simulink model "Simulation1"  (R2021a)
settings: Solver=VariableStepAuto  StartTime=0.0  StopTime=10.0  RelTol=1e-3
values from neighbouring files (symbols this model uses):
  Fp = 100    [ModelVisualisation.m]
  g = 9.81    [ModelVisualisation.m]    (also in Test.m)
  If = [Ixx 0 0;0 Iyy 0;0 0 Izz]    [ModelVisualisation.m]
  Kpm = mc/Ip    (= 0.005)    [ModelVisualisation.m]
  KVarianceBruit = 10    [ModelVisualisation.m]
  KVarianceBruiVent = 10    [ModelVisualisation.m]
  mi = 7    [ModelVisualisation.m]
  PhiRafale = pi/4    (= 0.785398163397)    [ModelVisualisation.m]
  Rafale = 5    [ModelVisualisation.m]
  SrefAA = LongueurAA*(CsaumonAA+CemplentureAA)/2    (= 0.02805)    [ModelVisualisation.m]
  SrefAC = LongueurAC*(CsaumonAC+CemplentureAC)/2    (= 0.002)    [ModelVisualisation.m]
  SrefC = 1/3*ZCC*2*pi*RayonCC    (= 0.0502654824574)    [ModelVisualisation.m]
  SrefCC = LongueurCC*pi*2*RayonCC    (= 1.25663706144)    [ModelVisualisation.m]
  TBruitP = 0.1    [ModelVisualisation.m]
  TBruitVent = 0.2    [ModelVisualisation.m]
  TDebutRafale = 2    [ModelVisualisation.m]
  TempsRafale = 0.7    [ModelVisualisation.m]
  Tpropultion = 2    [ModelVisualisation.m]
  VarianceBruitP = 1    [ModelVisualisation.m]
  VarianceBruitVent = 2    [ModelVisualisation.m]
settings Model: Creator=Adhemar  LastModifiedBy=adhem

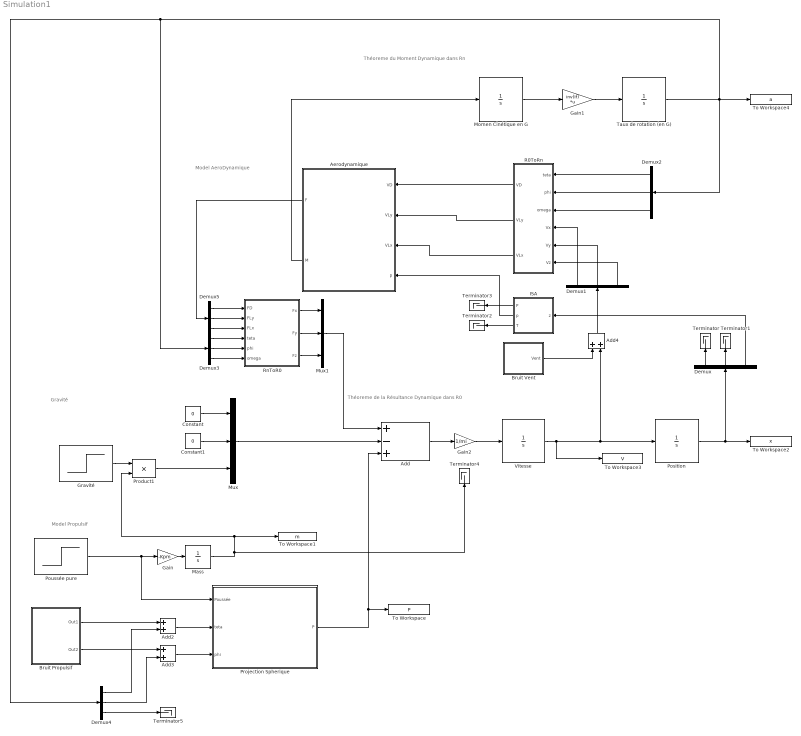
== system Simulation1 ==
  note: Théoreme du Moment Dynamique dans Rn
  note: Théoreme de la Résultance Dynamique dans R0
  note: Model AeroDynamique
  note: Gravité
  note: Model Propulsif
  Add : Sum  Inputs=+-+
  Add2 : Sum
  Add3 : Sum
  Add4 : Sum
  Aerodynamique : Subsystem
  Bruit Propulsif : Subsystem
  Bruit Vent : Subsystem
  Constant : Constant  Value=0
  Constant1 : Constant  Value=0
  Demux{,1..5} (6 alike) : Demux  Outputs=3
  Gain : Gain  Gain=-Kpm
  Gain1 : Gain  Gain=inv(If)  Multiplication=Matrix(K*u)
  Gain2 : Gain  Gain=1/mi
  Gravité : Step  Time=0  Before=g  After=g  SampleTime=0
  ISA : MATLAB Function  TreatAsAtomicUnit=on
  Mass : Integrator  InitialCondition=mi
  Momen Cinétique en G : Integrator
  Mux : Mux  Inputs=3
  Mux1 : Mux  Inputs=3
  Position : Integrator  InitialCondition=[0,0,0]
  Poussée pure : Step  Time=Tpropultion  Before=Fp  After=0  SampleTime=0
  Product1 : Product
  Projection Spherique : Subsystem
  R0ToRn : MATLAB Function  TreatAsAtomicUnit=on
  RnToR0 : MATLAB Function  TreatAsAtomicUnit=on
  Taux de rotation (en G) : Integrator
  Terminator{,1..5} (6 alike) : Terminator
  To Workspace : ToWorkspace  VariableName=P  SaveFormat=Timeseries  SampleTime=-1
  To Workspace1 : ToWorkspace  VariableName=m  SaveFormat=Timeseries  SampleTime=-1
  To Workspace2 : ToWorkspace  VariableName=x  SaveFormat=Timeseries  SampleTime=-1
  To Workspace3 : ToWorkspace  VariableName=V  SaveFormat=Timeseries  SampleTime=-1
  To Workspace4 : ToWorkspace  VariableName=a  SaveFormat=Timeseries  SampleTime=-1
  Vitesse : Integrator  InitialCondition=[0,0,0]
  wires:
  Add/1 -> Gain2/1
  Poussée pure/1 -> Gain/1, Projection Spherique/1(Poussée)
  Projection Spherique/1(P) -> Add/3, To Workspace/1
  Gravité/1 -> Product1/1
  Gain2/1 -> Vitesse/1
  Mass/1 -> Terminator4/1, To Workspace1/1, Product1/2
  Gain/1 -> Mass/1
  Product1/1 -> Mux/3
  Position/1 -> To Workspace2/1, Demux/1
  Bruit Propulsif/1(Out1) -> Add2/1
  Bruit Propulsif/2(Out2) -> Add3/1
  Mux1/1 -> Add/1
  Constant/1 -> Mux/1
  Mux/1 -> Add/2
  Constant1/1 -> Mux/2
  Demux/3 -> ISA/1(z)
  Demux/1 -> Terminator/1
  Demux/2 -> Terminator1/1
  Demux1/1 -> R0ToRn/4(Vx)
  Vitesse/1 -> Position/1, Add4/2, To Workspace3/1
  Demux1/3 -> R0ToRn/6(Vz)
  Demux1/2 -> R0ToRn/5(Vy)
  Momen Cinétique en G/1 -> Gain1/1
  Gain1/1 -> Taux de rotation (en G)/1
  Add2/1 -> Projection Spherique/2(teta)
  Add3/1 -> Projection Spherique/3(phi)
  Add4/1 -> Demux1/1
  Bruit Vent/1(Vent) -> Add4/1
  Demux2/3 -> R0ToRn/3(omega)
  Demux2/2 -> R0ToRn/2(phi)
  Demux2/1 -> R0ToRn/1(teta)
  RnToR0/1(Fx) -> Mux1/1
  RnToR0/2(Fy) -> Mux1/2
  RnToR0/3(Fz) -> Mux1/3
  Demux3/1 -> RnToR0/4(teta)
  Demux3/2 -> RnToR0/5(phi)
  Demux3/3 -> RnToR0/6(omega)
  Taux de rotation (en G)/1 -> Demux2/1, Demux4/1, Demux3/1, To Workspace4/1
  ISA/3(T) -> Terminator2/1
  ISA/1(P) -> Terminator3/1
  Demux4/1 -> Add2/2
  Demux4/2 -> Add3/2
  Demux4/3 -> Terminator5/1
  Aerodynamique/2(M) -> Momen Cinétique en G/1
  R0ToRn/1(VD) -> Aerodynamique/1(VD)
  R0ToRn/2(VLy) -> Aerodynamique/2(VLy)
  R0ToRn/3(VLx) -> Aerodynamique/3(VLx)
  ISA/2(p) -> Aerodynamique/4(p)
  Aerodynamique/1(F) -> Demux5/1
  Demux5/1 -> RnToR0/1(FD)
  Demux5/2 -> RnToR0/2(FLy)
  Demux5/3 -> RnToR0/3(FLx)

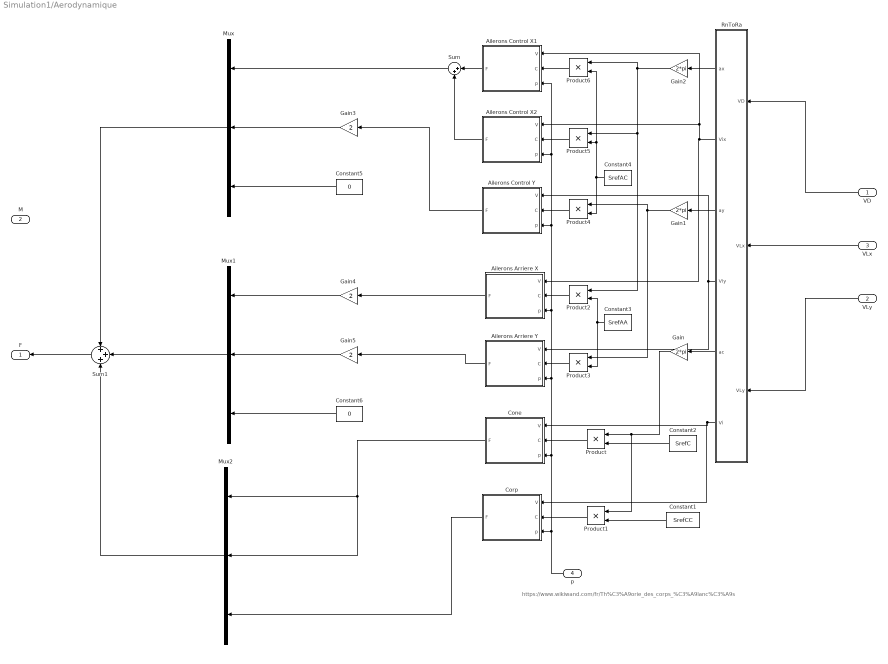
== system Simulation1/Aerodynamique ==
  note: https://www.wikiwand.com/fr/Th%C3%A9orie_des_corps_%C3%A9lanc%C3%A9s
  VD : Inport
  VLy : Inport  Port=2
  VLx : Inport  Port=3
  p : Inport  Port=4
  Ailerons Arriere X : MATLAB Function  TreatAsAtomicUnit=on
  Ailerons Arriere Y : MATLAB Function  TreatAsAtomicUnit=on
  Ailerons Control X1 : MATLAB Function  TreatAsAtomicUnit=on
  Ailerons Control X2 : MATLAB Function  TreatAsAtomicUnit=on
  Ailerons Control Y : MATLAB Function  TreatAsAtomicUnit=on
  Cone : MATLAB Function  TreatAsAtomicUnit=on
  Constant1 : Constant  Value=SrefCC
  Constant2 : Constant  Value=SrefC
  Constant3 : Constant  Value=SrefAA
  Constant4 : Constant  Value=SrefAC
  Constant5 : Constant  Value=0
  Constant6 : Constant  Value=0
  Corp : MATLAB Function  TreatAsAtomicUnit=on
  Gain : Gain  Gain=2*pi
  Gain1 : Gain  Gain=2*pi
  Gain2 : Gain  Gain=2*pi
  Gain3 : Gain  Gain=2
  Gain4 : Gain  Gain=2
  Gain5 : Gain  Gain=2
  Mux : Mux  Inputs=3
  Mux1 : Mux  Inputs=3
  Mux2 : Mux  Inputs=3
  Product{,1..6} (7 alike) : Product
  RnToRa : MATLAB Function  TreatAsAtomicUnit=on
  Sum : Sum  Inputs=|++
  Sum1 : Sum  Inputs=+++
  F : Outport
  M : Outport  Port=2
  wires:
  VLy/1 -> RnToRa/3(VLy)
  p/1 -> Ailerons Control Y/3(p), Ailerons Control X2/3(p), Ailerons Control X1/3(p), Ailerons Arriere X/3(p), Ailerons Arriere Y/3(p), Cone/3(p), Corp/3(p)
  Constant2/1 -> Product/2
  Corp/1(F) -> Mux2/3
  VLx/1 -> RnToRa/2(VLx)
  VD/1 -> RnToRa/1(VD)
  Ailerons Arriere X/1(F) -> Gain4/1
  Cone/1(F) -> Mux2/2, Mux2/1
  RnToRa/1(ax) -> Gain2/1
  RnToRa/5(ac) -> Gain/1
  Gain/1 -> Product1/1, Product/1
  Product/1 -> Cone/2(C)
  Constant1/1 -> Product1/2
  Product1/1 -> Corp/2(C)
  RnToRa/6(Vi) -> Cone/1(V), Corp/1(V)
  RnToRa/3(ay) -> Gain1/1
  Gain2/1 -> Product5/1, Product2/1, Product6/1
  Product2/1 -> Ailerons Arriere X/2(C)
  Product3/1 -> Ailerons Arriere Y/2(C)
  Gain1/1 -> Product3/1, Product4/1
  Constant3/1 -> Product2/2, Product3/2
  Product4/1 -> Ailerons Control Y/2(C)
  Product5/1 -> Ailerons Control X2/2(C)
  Product6/1 -> Ailerons Control X1/2(C)
  Constant4/1 -> Product5/2, Product6/2, Product4/2
  Sum/1 -> Mux/1
  Ailerons Control X1/1(F) -> Sum/1
  Ailerons Control X2/1(F) -> Sum/2
  Ailerons Control Y/1(F) -> Gain3/1
  Gain3/1 -> Mux/2
  Constant5/1 -> Mux/3
  Gain4/1 -> Mux1/1
  Constant6/1 -> Mux1/3
  Ailerons Arriere Y/1(F) -> Gain5/1
  Gain5/1 -> Mux1/2
  RnToRa/4(Viy) -> Ailerons Control Y/1(V), Ailerons Arriere Y/1(V)
  RnToRa/2(Vix) -> Ailerons Arriere X/1(V), Ailerons Control X1/1(V), Ailerons Control X2/1(V)
  Sum1/1 -> F/1
  Mux1/1 -> Sum1/2
  Mux2/1 -> Sum1/3
  Mux/1 -> Sum1/1

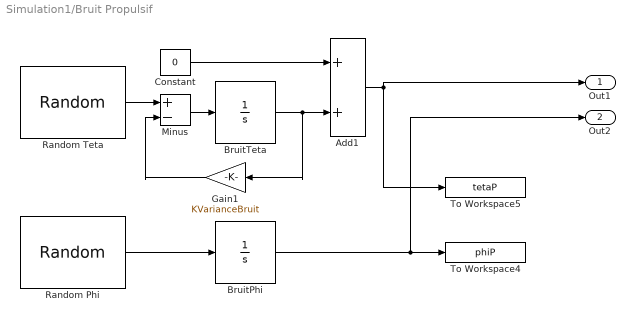
== system Simulation1/Bruit Propulsif ==
  Add1 : Sum
  BruitPhi : Integrator
  BruitTeta : Integrator
  Constant : Constant  Value=0
  Gain1 : Gain  Gain=KVarianceBruit
  Minus : Sum  Inputs=+-
  Random Phi : RandomNumber  Variance=VarianceBruitP  SampleTime=TBruitP
  Random Teta : RandomNumber  Variance=VarianceBruitP  Seed=1  SampleTime=TBruitP
  To Workspace4 : ToWorkspace  VariableName=phiP  SaveFormat=Timeseries  SampleTime=-1
  To Workspace5 : ToWorkspace  VariableName=tetaP  SaveFormat=Timeseries  SampleTime=-1
  Out1 : Outport
  Out2 : Outport  Port=2
  wires:
  Minus/1 -> BruitTeta/1
  BruitPhi/1 -> Out2/1, To Workspace4/1
  BruitTeta/1 -> Gain1/1, Add1/2
  Random Phi/1 -> BruitPhi/1
  Add1/1 -> Out1/1, To Workspace5/1
  Random Teta/1 -> Minus/1
  Gain1/1 -> Minus/2
  Constant/1 -> Add1/1

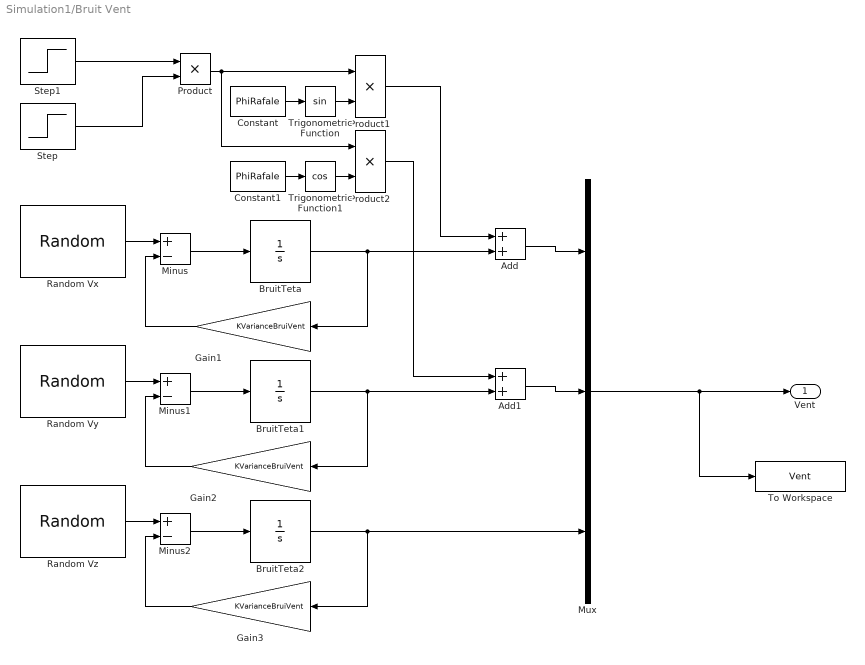
== system Simulation1/Bruit Vent ==
  Add : Sum
  Add1 : Sum
  BruitTeta : Integrator
  BruitTeta1 : Integrator
  BruitTeta2 : Integrator
  Constant : Constant  Value=PhiRafale
  Constant1 : Constant  Value=PhiRafale
  Gain1 : Gain  Gain=KVarianceBruiVent
  Gain2 : Gain  Gain=KVarianceBruiVent
  Gain3 : Gain  Gain=KVarianceBruiVent
  Minus : Sum  Inputs=+-
  Minus1 : Sum  Inputs=+-
  Minus2 : Sum  Inputs=+-
  Mux : Mux  Inputs=3
  Product : Product
  Product1 : Product
  Product2 : Product
  Random Vx : RandomNumber  Variance=VarianceBruitVent  SampleTime=TBruitVent
  Random Vy : RandomNumber  Variance=VarianceBruitVent  Seed=1  SampleTime=TBruitVent
  Random Vz : RandomNumber  Variance=VarianceBruitVent  Seed=2  SampleTime=TBruitVent
  Step : Step  Time=TDebutRafale  After=Rafale  SampleTime=0
  Step1 : Step  Time=TDebutRafale+TempsRafale  Before=1  After=0  SampleTime=0
  To Workspace : ToWorkspace  VariableName=Vent  SaveFormat=Timeseries  SampleTime=-1
  Trigonometric Function : Trigonometry
  Trigonometric Function1 : Trigonometry  Operator=cos
  Vent : Outport
  wires:
  Minus/1 -> BruitTeta/1
  BruitTeta/1 -> Add/2, Gain1/1
  Random Vx/1 -> Minus/1
  Gain1/1 -> Minus/2
  Mux/1 -> To Workspace/1, Vent/1
  Gain2/1 -> Minus1/2
  Minus1/1 -> BruitTeta1/1
  BruitTeta1/1 -> Add1/2, Gain2/1
  Random Vy/1 -> Minus1/1
  Minus2/1 -> BruitTeta2/1
  Random Vz/1 -> Minus2/1
  Gain3/1 -> Minus2/2
  BruitTeta2/1 -> Mux/3, Gain3/1
  Step/1 -> Product/2
  Step1/1 -> Product/1
  Product/1 -> Product2/1, Product1/1
  Add/1 -> Mux/1
  Product1/1 -> Add/1
  Trigonometric Function/1 -> Product1/2
  Constant/1 -> Trigonometric Function/1
  Add1/1 -> Mux/2
  Constant1/1 -> Trigonometric Function1/1
  Trigonometric Function1/1 -> Product2/2
  Product2/1 -> Add1/1

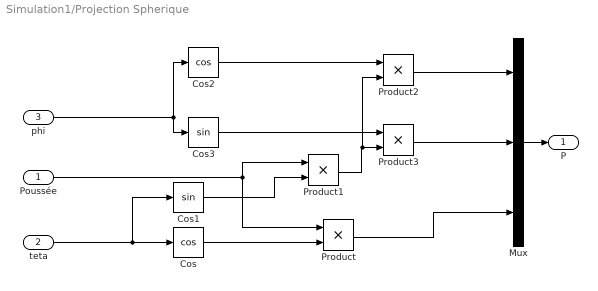
== system Simulation1/Projection Spherique ==
  Poussée : Inport
  teta : Inport  Port=2
  phi : Inport  Port=3
  Cos : Trigonometry  Operator=cos
  Cos1 : Trigonometry
  Cos2 : Trigonometry  Operator=cos
  Cos3 : Trigonometry
  Mux : Mux  Inputs=3
  Product{,1..3} (4 alike) : Product
  P : Outport
  wires:
  Poussée/1 -> Product1/1, Product/1
  Cos/1 -> Product/2
  teta/1 -> Cos1/1, Cos/1
  Product/1 -> Mux/3
  Cos1/1 -> Product1/2
  phi/1 -> Cos3/1, Cos2/1
  Product2/1 -> Mux/1
  Product3/1 -> Mux/2
  Product1/1 -> Product2/2, Product3/2
  Cos3/1 -> Product3/1
  Cos2/1 -> Product2/1
  Mux/1 -> P/1

== matlab function Simulation1/Aerodynamique/Ailerons Arriere Y ==
  data: V input; C input; p input; F output
function F = VToFAero(V,C,p)
    F=0.5*p*C*V^2;
end

== matlab function Simulation1/Aerodynamique/Ailerons Control X2 ==
  data: V input; C input; p input; F output
function F = VToFAero(V,C,p)
    F=0.5*p*C*V^2;
end

== matlab function Simulation1/Aerodynamique/Ailerons Control Y ==
  data: V input; C input; p input; F output
function F = VToFAero(V,C,p)
    F=0.5*p*C*V^2;
end

== matlab function Simulation1/R0ToRn ==
  data: teta input; phi input; omega input; Vx input; VD output; VLy output; Vy input; Vz input; VLx output
function [VD,VLy,VLx] = ChangementBase(teta,phi,omega,Vx,Vy,Vz)
    V=sqrt(Vx^2+Vy^2+Vz^2);
    
    %Changement base B
    VBx=cos(phi)*Vx+sin(phi)*Vy;
    VBy=cos(phi)*Vy-sin(phi)*Vx;
    VBz=Vz;
    %Changement base A
    VAx=VBx;
    VAy=cos(teta)*VBy+sin(teta)*VBz;
    VAz=cos(teta)*VBz-sin(teta)*VBy;
    %Changement base Aérodynamique
    VD=VAz;
    VLx=VAx*cos(omega)+VAy*sin(omega);
    VLy=VAy*cos(omega)-VAx*sin(omega);
    
    
    
    % A faire sous forme de matrice de passage
end

== matlab function Simulation1/ISA ==
  data: z input; P output; p output; T output

function [P,p,T]=ISA(z)
    
    g=9.81;
    r=287.04; %Constante des gaz parfait air (J/Kg/K)
    T0=287.15; %Température au sol A regler avant le lancement (K)
    Tz=-0.0065; %(K)
    P0=101325; %Pression au sol à regler avant le lancement (pa)
    p0=P0/(r*T0); %Densité de l'air (Kg/m3) 
    
    T=double(T0+Tz*z);
    P=double(P0*(1+(Tz/T0)*z)^(-g/(r*Tz)));
    p=double(P/(r*T));
end

== matlab function Simulation1/RnToR0 ==
  data: FD input; Fx output; FLy input; FLx input; teta input; phi input; omega input; Fy output; Fz output
function [Fx,Fy,Fz] = ChangeBase(FD,FLy,FLx,teta,phi,omega)
    Fx=0;
    Fy=0;
    Fz=0;
end

== matlab function Simulation1/Aerodynamique/Cone ==
  data: V input; C input; p input; F output
function F = VToFAero(V,C,p)
    F=0.5*p*C*V^2;
end

== matlab function Simulation1/Aerodynamique/Corp ==
  data: V input; C input; p input; F output
function F = VToFAero(V,C,p)
    F=0.5*p*C*V^2;
end

== matlab function Simulation1/Aerodynamique/Ailerons Arriere X ==
  data: V input; C input; p input; F output
function F = VToFAero(V,C,p)
    F=0.5*p*C*V^2;
end

== matlab function Simulation1/Aerodynamique/Ailerons Control X1 ==
  data: V input; C input; p input; F output
function F = VToFAero(V,C,p)
    F=0.5*p*C*V^2;
end

== matlab function Simulation1/Aerodynamique/RnToRa ==
  data: VD input; ax output; VLx input; VLy input; Vix output; ay output; Viy output; ac output; Vi output
function [ax,Vix,ay,Viy,ac,Vi] = ChangeBase(VD,VLx,VLy)
    
    ax=atan(VLx/VD);
    Vix=sqrt(VD^2+VLx^2)
    
    ay=atan(VLy/VD);
    Viy=sqrt(VD^2+VLy^2)
    
    ac=atan(sqrt(VLx^2+VLy^2)/VD)
    Vi=sqrt(VD^2+VLx^2+VLy^2)
end
